simulink model "x12_foc_iden_Jx"  (R2023b)
settings: Solver=VariableStepAuto  StartTime=0.0  StopTime=1  RelTol=1e-3
values from neighbouring files (symbols this model uses):
  Fcoef = 0    [foc_para.m]
  Flux = 0.00525    [foc_para.m]
  id_ki = Rs*CurrentLoopBandwidth    (= 1413.71669412)    [foc_para.m]
  id_kp = Ls*CurrentLoopBandwidth    (= 1.31946891451)    [foc_para.m]
  iq_ki = Rs*CurrentLoopBandwidth    (= 1413.71669412)    [foc_para.m]
  iq_kp = Ls*CurrentLoopBandwidth    (= 1.31946891451)    [foc_para.m]
  iq_limit = 50    [foc_para.m]
  Jx = 0.000004483738    (= 4.483738e-06)    [foc_para.m]
  Ls = 0.00042    [foc_para.m]
  Np = 4    [foc_para.m]
  spd_ki = ((iq_kp/Ls)*(iq_kp/Ls))/(delta*delta*delta*K)    (= 43.9015082323)    [foc_para.m]
  spd_kp = (iq_kp/Ls)/(delta*K)/9.55    (= 0.0234124131329)    [foc_para.m]
  Tpwm = 4000-1    (= 3999)    [foc_para.m]
  Ts = 1/SwitchFrequency    (= 5e-05)    [foc_para.m]
  vbus = 24    [foc_para.m]
  vd_limit = vbus/sqrt(3)    [foc_para.m]
  vq_limit = vbus/sqrt(3)    [foc_para.m]
undefined symbols (not defined in the file or in its folder): DiscIntNeverNeededParam
libraries: spsMosfetLib x6, simulink x3, spsVoltageMeasurementLib x3, spsPermanentMagnetSynchronousMachineLib x1, spsDCVoltageSourceLib x1, sps_lib x1
settings Model: Creator=disnox  LastModifiedBy=disno
settings DataIOCC: ReturnWorkspaceOutputs=off
settings DebuggingCC: ParameterPrecisionLossMsg=none

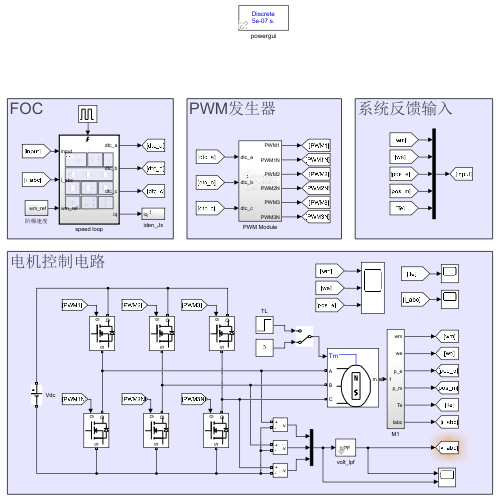
[thumbnail: Simulink's stored preview of the top-level diagram]
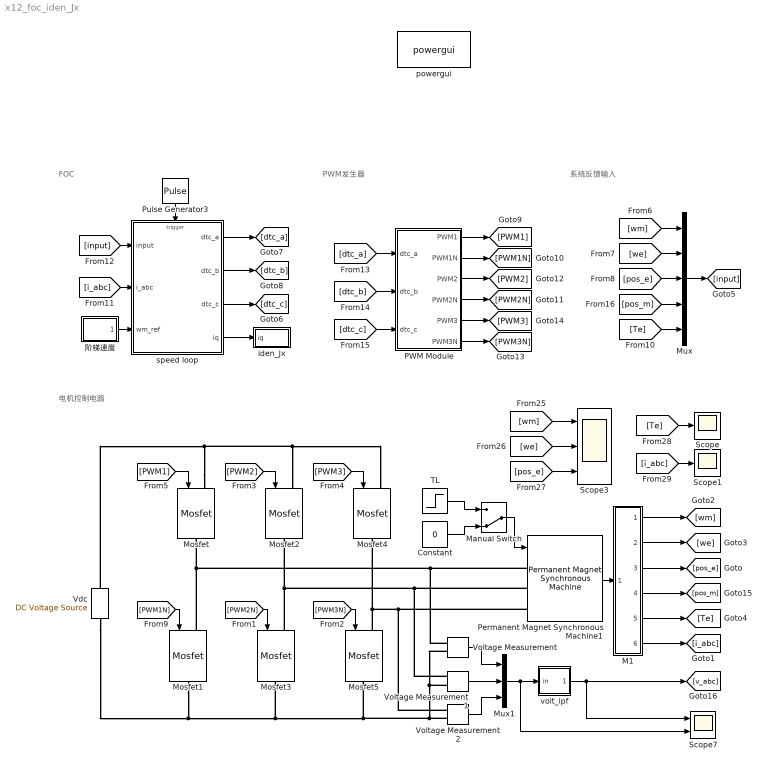
== system x12_foc_iden_Jx ==
  note: FOC
  note: PWM发生器
  note: 系统反馈输入
  note: 电机控制电路
  Constant : Constant  Value=0
  M1 : Subsystem
  Manual Switch : ManualSwitch  CurrentSetting=0
  Mosfet{,1..5} (6 alike) : spsMosfetLib/Mosfet  Ron=0.1  Lon=0  Rd=0.01  Vfd=0  IC=0  Rs=1e5  Cs=inf  Measurements=off
  Mux : Mux  Inputs=5
  Mux1 : Mux  Inputs=3
  PWM Module : Subsystem
  Permanent Magnet Synchronous Machine1 : spsPermanentMagnetSynchronousMachineLib/Permanent Magnet Synchronous Machine  NbPhases=3  FluxDistribution=Sinusoidal  RotorType=Salient-pole  MechanicalLoad=Torque Tm  PresetModel=No  ShowDetailedParameters=on  MeasurementBus=off  Resistance=(Rs)  Inductance=8.5e-3  dqInductances=[Ls, Ls]  La=0.000835  MachineConstant=Flux linkage established by magnets (V.s)  Flux=Flux  VoltageCst=3.809  TorqueCst=0.0315  Flat=120  Mechanical=[Jx Fcoef Np 0]  PolePairs=Np  InitialConditions=[0,0, 0,0]  InitialConditions5ph=[0 0 0 0 0 0]  RefAngle=Aligned with phase A axis (original Park)  IterativeDiscreteModel=Trapezoidal non iterative  TsBlock=-1  TsPowergui=0
  Pulse Generator3 : DiscretePulseGenerator  PulseType=Time based  Period=Ts  PulseWidth=50
  Scope : Scope
  Scope1 : Scope
  Scope3 : Scope  NumInputPorts=3
  Scope7 : Scope  NumInputPorts=2
  TL : Step  Time=0.1  After=0.05  SampleTime=0
  Vdc : spsDCVoltageSourceLib/DC Voltage Source  Amplitude=vbus  Measurements=None
  Voltage Measurement : spsVoltageMeasurementLib/Voltage Measurement  PhasorSimulation=off  OutputType=Complex  PSBequivalent=0
  Voltage Measurement1 : spsVoltageMeasurementLib/Voltage Measurement  PhasorSimulation=off  OutputType=Complex  PSBequivalent=0
  Voltage Measurement2 : spsVoltageMeasurementLib/Voltage Measurement  PhasorSimulation=off  OutputType=Complex  PSBequivalent=0
  iden_Jx : Subsystem
  powergui : sps_lib/powergui  SimulationMode=Discrete  SampleTime=Ts/100  frequency=60  Iterations=50  frequencyindice=0  Pbase=100e6  ErrMax=1e-4  UnitsV=kV  UnitsW=MW  buscounter=0  FunctionMessages=off  echomessages=off  EnableUseOfTLC=off  CurrentSourceSwitches=off  DisableSnubberDevices=off  DisableRonSwitches=off  DisableVfSwitches=off  DisplayEquations=off  AutomaticDiscreteSolvers=off  SolverType=Tustin/Backward Euler (TBE)  Interpol=off  ExternalGateDelay=off  methode=off  Ts=0  x0status=blocks  SPID=off  SwTol=0  HookPort=off  NonlinearTolerance=1e-4  nMaxIteration=100  ContinueOnMaxIteration=off  RestoreLinks=warning  ResistiveCurrentMeasurement=off  Frange=[0:2:500]  Ylog=off  Xlog=on  ShowGrid=off  save=off  variable=ZData  structure=0  ZoomFFT=off  StartTime=0.0  cycles=1  DisplayStyle=1  fundamental=60  FreqAxis=off  MaxFrequency=1000  frequencyindicesteady=1  RmsSteady=1  display=off
  speed loop : Subsystem
  volt_lpf : Subsystem  mask{lpf_freq=1000, Ts=Ts/100}
      mask DialogControl ParameterGroupVar Prompt: 参数
      mask Display: disp('LPF')
  阶梯速度 : Subsystem
  wires:
  Pulse Generator3/1 -> speed loop/Trigger
  [input] -> speed loop/1(input)
  speed loop/2(dtc_b) -> [dtc_b]
  speed loop/1(dtc_a) -> [dtc_a]
  speed loop/3(dtc_c) -> [dtc_c]
  [dtc_a] -> PWM Module/1(dtc_a)
  [dtc_b] -> PWM Module/2(dtc_b)
  [dtc_c] -> PWM Module/3(dtc_c)
  PWM Module/1(PWM1) -> [PWM1]
  PWM Module/2(PWM1N) -> [PWM1N]
  PWM Module/3(PWM2) -> [PWM2]
  PWM Module/4(PWM2N) -> [PWM2N]
  PWM Module/5(PWM3) -> [PWM3]
  PWM Module/6(PWM3N) -> [PWM3N]
  [i_abc] -> speed loop/2(i_abc)
  Mux/1 -> [input]
  [Te] -> Mux/5
  [pos_m] -> Mux/4
  [pos_e] -> Mux/3
  [we] -> Mux/2
  [wm] -> Mux/1
  Manual Switch/1 -> Permanent Magnet Synchronous Machine1/1
  TL/1 -> Manual Switch/1
  [PWM1] -> Mosfet/1
  [PWM2] -> Mosfet2/1
  Constant/1 -> Manual Switch/2
  [PWM2N] -> Mosfet3/1
  Mux1/1 -> Scope7/2, volt_lpf/1(in)
  [PWM3N] -> Mosfet5/1
  M1/1(wm) -> [wm]
  volt_lpf/1(out) -> Scope7/1, [v_abc]
  [PWM3] -> Mosfet4/1
  Voltage Measurement1/1 -> Mux1/2
  [we] -> Scope3/2
  [Te] -> Scope/1
  [pos_e] -> Scope3/3
  Permanent Magnet Synchronous Machine1/1 -> M1/1(In1)
  [wm] -> Scope3/1
  [i_abc] -> Scope1/1
  M1/4(p_m) -> [pos_m]
  Voltage Measurement/1 -> Mux1/1
  M1/6(Iabc) -> [i_abc]
  Voltage Measurement2/1 -> Mux1/3
  [PWM1N] -> Mosfet1/1
  M1/2(we) -> [we]
  M1/3(p_e) -> [pos_e]
  M1/5(Te) -> [Te]
  阶梯速度/1(wm_ref) -> speed loop/3(wm_ref)
  speed loop/4(iq) -> iden_Jx/1(iq)
  connections:
  Voltage Measurement2/LConn1 -- Mosfet5/LConn1 -- Mosfet4/RConn1 -- Permanent Magnet Synchronous Machine1/LConn3
  Mosfet3/RConn1 -- Voltage Measurement2/LConn2 -- Voltage Measurement1/LConn2 -- Voltage Measurement/LConn2 -- Mosfet5/RConn1 -- Vdc/LConn1 -- Mosfet1/RConn1
  Voltage Measurement/LConn1 -- Mosfet1/LConn1 -- Mosfet/RConn1 -- Permanent Magnet Synchronous Machine1/LConn1
  Mosfet/LConn1 -- Mosfet2/LConn1 -- Mosfet4/LConn1 -- Vdc/RConn1
  Mosfet2/RConn1 -- Mosfet3/LConn1 -- Permanent Magnet Synchronous Machine1/LConn2 -- Voltage Measurement1/LConn1

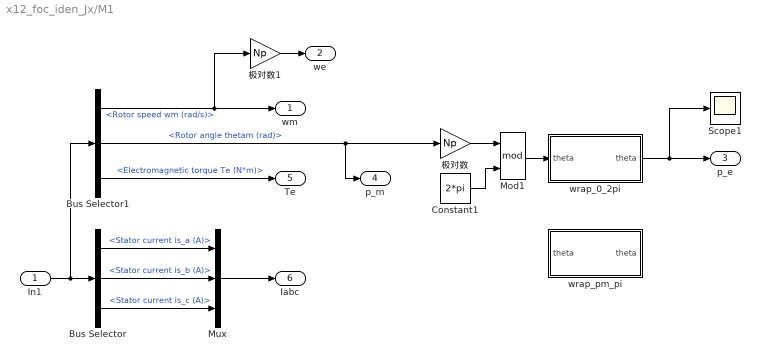
== system x12_foc_iden_Jx/M1 ==
  In1 : Inport
  Bus Selector : BusSelector  OutputSignals=Stator current is_a (A),Stator current is_b (A),Stator current is_c (A)
  Bus Selector1 : BusSelector  OutputSignals=Rotor speed wm (rad/s),Rotor angle thetam (rad),Electromagnetic torque Te (N*m)
  Constant1 : Constant  Value=2*pi
  Mod1 : Math  Operator=mod
  Mux : Mux  Inputs=3
  Scope1 : Scope
  wrap_0_2pi : MATLAB Function  TreatAsAtomicUnit=on
  wrap_pm_pi : MATLAB Function  TreatAsAtomicUnit=on
  极对数 : Gain  Gain=Np
  极对数1 : Gain  Gain=Np
  wm : Outport
  we : Outport  Port=2
  p_e : Outport  Port=3
  p_m : Outport  Port=4
  Te : Outport  Port=5
  Iabc : Outport  Port=6
  wires:
  Bus Selector/1 -> Mux/1  "<Stator current is_a (A)>"
  Bus Selector/2 -> Mux/2  "<Stator current is_b (A)>"
  Bus Selector/3 -> Mux/3  "<Stator current is_c (A)>"
  Bus Selector1/1 -> 极对数1/1, wm/1  "<Rotor speed wm (rad/s)>"
  Bus Selector1/2 -> p_m/1, 极对数/1  "<Rotor angle thetam (rad)>"
  Bus Selector1/3 -> Te/1  "<Electromagnetic torque Te (N*m)>"
  Mux/1 -> Iabc/1
  In1/1 -> Bus Selector1/1, Bus Selector/1
  Constant1/1 -> Mod1/2
  极对数/1 -> Mod1/1
  Mod1/1 -> wrap_0_2pi/1("theta ")
  wrap_0_2pi/1(theta) -> Scope1/1, p_e/1
  极对数1/1 -> we/1

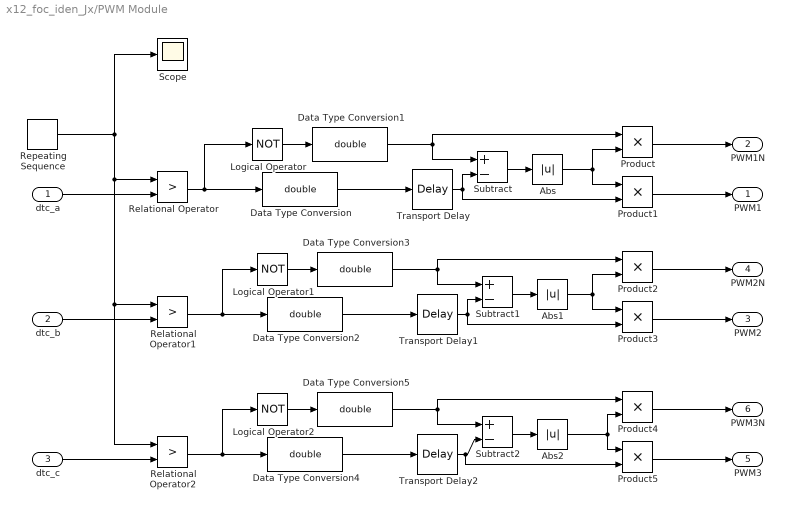
== system x12_foc_iden_Jx/PWM Module ==
  dtc_a : Inport
  dtc_b : Inport  Port=2
  dtc_c : Inport  Port=3
  Abs : Abs  SaturateOnIntegerOverflow=off
  Abs1 : Abs  SaturateOnIntegerOverflow=off
  Abs2 : Abs  SaturateOnIntegerOverflow=off
  Data Type Conversion{,1..5} (6 alike) : DataTypeConversion  OutDataTypeStr=double  SaturateOnIntegerOverflow=off  RndMeth=Floor
  Logical Operator : Logic  Operator=NOT  AllPortsSameDT=off  OutDataTypeStr=boolean
  Logical Operator1 : Logic  Operator=NOT  AllPortsSameDT=off  OutDataTypeStr=boolean
  Logical Operator2 : Logic  Operator=NOT  AllPortsSameDT=off  OutDataTypeStr=boolean
  Product{,1..5} (6 alike) : Product
  Relational Operator : RelationalOperator  Operator=>  OutDataTypeStr=boolean  RndMeth=Simplest  InputSameDT=off
  Relational Operator1 : RelationalOperator  Operator=>  OutDataTypeStr=boolean  RndMeth=Simplest  InputSameDT=off
  Relational Operator2 : RelationalOperator  Operator=>  OutDataTypeStr=boolean  RndMeth=Simplest  InputSameDT=off
  Repeating Sequence : simulink/Sources/Repeating Sequence  rep_seq_t=[0 Ts/2 Ts]  rep_seq_y=[0 Tpwm 0]
  Scope : Scope
  Subtract : Sum  Inputs=+-
  Subtract1 : Sum  Inputs=+-
  Subtract2 : Sum  Inputs=+-
  Transport Delay : TransportDelay  DelayTime=168/168e6
  Transport Delay1 : TransportDelay  DelayTime=168/168e6
  Transport Delay2 : TransportDelay  DelayTime=168/168e6
  PWM1 : Outport
  PWM1N : Outport  Port=2
  PWM2 : Outport  Port=3
  PWM2N : Outport  Port=4
  PWM3 : Outport  Port=5
  PWM3N : Outport  Port=6
  wires:
  Product1/1 -> PWM1/1
  Relational Operator1/1 -> Logical Operator1/1, Data Type Conversion2/1
  Logical Operator2/1 -> Data Type Conversion5/1
  Subtract/1 -> Abs/1
  Relational Operator2/1 -> Data Type Conversion4/1, Logical Operator2/1
  Product4/1 -> PWM3N/1
  Data Type Conversion5/1 -> Subtract2/1, Product4/1
  Product2/1 -> PWM2N/1
  Abs1/1 -> Product2/2, Product3/1
  Transport Delay2/1 -> Subtract2/2, Product5/2
  Repeating Sequence/1 -> Scope/1, Relational Operator/1, Relational Operator2/1, Relational Operator1/1
  Data Type Conversion/1 -> Transport Delay/1
  Product/1 -> PWM1N/1
  Product3/1 -> PWM2/1
  Abs2/1 -> Product5/1, Product4/2
  Data Type Conversion2/1 -> Transport Delay1/1
  dtc_a/1 -> Relational Operator/2
  Transport Delay/1 -> Product1/2, Subtract/2
  Subtract1/1 -> Abs1/1
  Data Type Conversion3/1 -> Subtract1/1, Product2/1
  dtc_c/1 -> Relational Operator2/2
  Logical Operator/1 -> Data Type Conversion1/1
  Transport Delay1/1 -> Product3/2, Subtract1/2
  Relational Operator/1 -> Logical Operator/1, Data Type Conversion/1
  Abs/1 -> Product/2, Product1/1
  Product5/1 -> PWM3/1
  Data Type Conversion4/1 -> Transport Delay2/1
  Subtract2/1 -> Abs2/1
  Logical Operator1/1 -> Data Type Conversion3/1
  Data Type Conversion1/1 -> Subtract/1, Product/1
  dtc_b/1 -> Relational Operator1/2

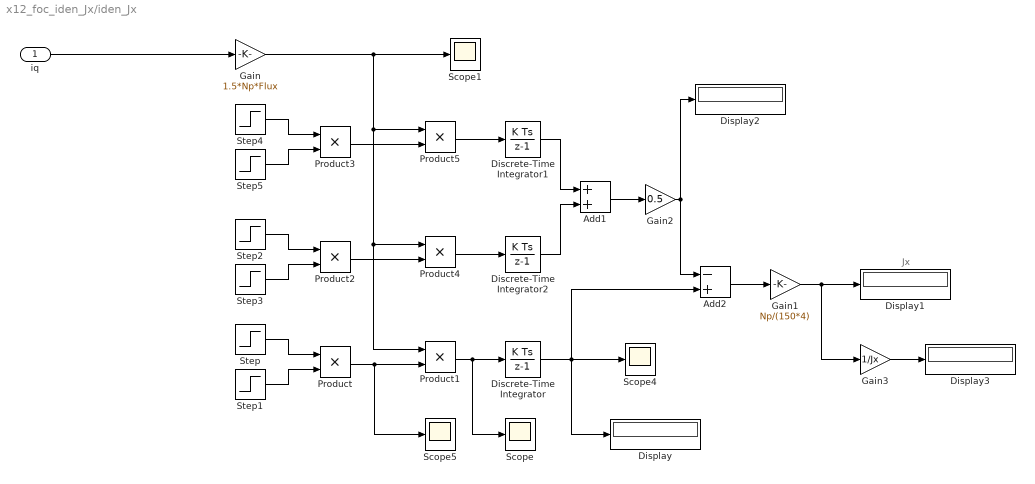
== system x12_foc_iden_Jx/iden_Jx ==
  note: Jx
  iq : Inport
  Add1 : Sum
  Add2 : Sum  Inputs=-+
  Discrete-Time Integrator : DiscreteIntegrator  SampleTime=-1  ICPrevOutput=DiscIntNeverNeededParam  ICPrevScaledInput=DiscIntNeverNeededParam
  Discrete-Time Integrator1 : DiscreteIntegrator  SampleTime=-1  ICPrevOutput=DiscIntNeverNeededParam  ICPrevScaledInput=DiscIntNeverNeededParam
  Discrete-Time Integrator2 : DiscreteIntegrator  SampleTime=-1  ICPrevOutput=DiscIntNeverNeededParam  ICPrevScaledInput=DiscIntNeverNeededParam
  Display{,1..3} (4 alike) : Display
  Gain : Gain  Gain=1.5*Np*Flux
  Gain1 : Gain  Gain=Np/(150*4)
  Gain2 : Gain  Gain=0.5
  Gain3 : Gain  Gain=1/Jx
  Product{,1..5} (6 alike) : Product
  Scope{,1,4..5} (4 alike) : Scope
  Step : Step  Time=0.65  SampleTime=0
  Step1 : Step  Time=0.8  Before=1  After=0  SampleTime=0
  Step2 : Step  Time=0.83  SampleTime=0
  Step3 : Step  Time=0.98  Before=1  After=0  SampleTime=0
  Step4 : Step  Time=0.42  SampleTime=0
  Step5 : Step  Time=0.57  Before=1  After=0  SampleTime=0
  wires:
  Step4/1 -> Product3/1
  Product/1 -> Scope5/1, Product1/2
  Product3/1 -> Product5/2
  Gain/1 -> Scope1/1, Product5/1, Product4/1, Product1/1
  Step1/1 -> Product/2
  Product1/1 -> Scope/1, Discrete-Time Integrator/1
  Product2/1 -> Product4/2
  Gain2/1 -> Display2/1, Add2/1
  Step/1 -> Product/1
  Discrete-Time Integrator1/1 -> Add1/1
  Step5/1 -> Product3/2
  Step3/1 -> Product2/2
  Discrete-Time Integrator/1 -> Scope4/1, Display/1, Add2/2
  Step2/1 -> Product2/1
  Product5/1 -> Discrete-Time Integrator1/1
  Add1/1 -> Gain2/1
  Discrete-Time Integrator2/1 -> Add1/2
  Add2/1 -> Gain1/1
  Gain1/1 -> Gain3/1, Display1/1
  Product4/1 -> Discrete-Time Integrator2/1
  iq/1 -> Gain/1
  Gain3/1 -> Display3/1

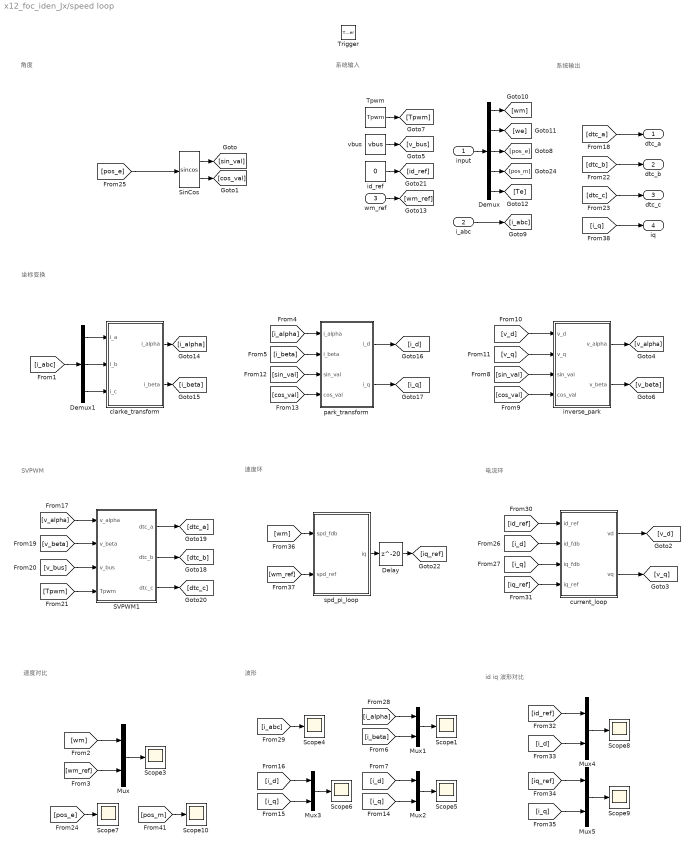
== system x12_foc_iden_Jx/speed loop ==
  note: 角度
  note: 坐标变换
  note: SVPWM
  note: 速度对比
  note: 波形
  note: 系统输入
  note: 系统输出
  note: 电流环
  note: id iq 波形对比
  note: 速度环
  input : Inport
  i_abc : Inport  Port=2
  wm_ref : Inport  Port=3
  Trigger : TriggerPort  VariantControl=(inherit)
  Delay : Delay  DelayLength=20
  Demux : Demux  Outputs=5
  Demux1 : Demux  Outputs=3
  Mux{,1..5} (6 alike) : Mux  Inputs=2
  SVPWM1 : Subsystem  TreatAsAtomicUnit=on
      settings: RTWSystemCode=Nonreusable function  RTWFcnNameOpts=Use subsystem name
  Scope{1,3..10} (9 alike) : Scope
  SinCos : Trigonometry  Operator=sincos
  Tpwm : Constant  Value=Tpwm
  clarke_transform : Subsystem  TreatAsAtomicUnit=on
      settings: RTWSystemCode=Nonreusable function  RTWFcnNameOpts=Use subsystem name
  current_loop : Subsystem
  id_ref : Constant  Value=0
  inverse_park : Subsystem  TreatAsAtomicUnit=on
      settings: RTWSystemCode=Nonreusable function  RTWFcnNameOpts=Use subsystem name
  park_transform : Subsystem  TreatAsAtomicUnit=on
      settings: RTWSystemCode=Nonreusable function  RTWFcnNameOpts=Use subsystem name
  spd_pi_loop : Subsystem  TreatAsAtomicUnit=on
      settings: RTWSystemCode=Nonreusable function  RTWFcnNameOpts=Use subsystem name
  vbus : Constant  Value=vbus
  dtc_a : Outport
  dtc_b : Outport  Port=2
  dtc_c : Outport  Port=3
  iq : Outport  Port=4
  wires:
  SinCos/1 -> [sin_val]
  SinCos/2 -> [cos_val]
  wm_ref/1 -> [wm_ref]
  id_ref/1 -> [id_ref]
  [cos_val] -> inverse_park/4(cos_val)
  [sin_val] -> park_transform/3(sin_val)
  [v_d] -> inverse_park/1(v_d)
  [v_q] -> inverse_park/2(v_q)
  [cos_val] -> park_transform/4(cos_val)
  [sin_val] -> inverse_park/3(sin_val)
  [v_beta] -> SVPWM1/2(v_beta)
  [v_alpha] -> SVPWM1/1(v_alpha)
  [Tpwm] -> SVPWM1/4(Tpwm)
  [v_bus] -> SVPWM1/3(v_bus)
  Tpwm/1 -> [Tpwm]
  vbus/1 -> [v_bus]
  inverse_park/2(v_beta) -> [v_beta]
  inverse_park/1(v_alpha) -> [v_alpha]
  Demux1/1 -> clarke_transform/1(i_a)
  Demux1/2 -> clarke_transform/2(i_b)
  Demux1/3 -> clarke_transform/3(i_c)
  [i_abc] -> Demux1/1
  [wm] -> Mux/1
  [wm_ref] -> Mux/2
  Mux/1 -> Scope3/1
  i_abc/1 -> [i_abc]
  [i_alpha] -> park_transform/1(i_alpha)
  [i_beta] -> park_transform/2(i_beta)
  clarke_transform/1(i_alpha) -> [i_alpha]
  clarke_transform/2(i_beta) -> [i_beta]
  park_transform/1(i_d) -> [i_d]
  park_transform/2(i_q) -> [i_q]
  [i_abc] -> Scope4/1
  [i_alpha] -> Mux1/1
  Mux1/1 -> Scope1/1
  [i_beta] -> Mux1/2
  [i_q] -> Mux2/2
  [i_d] -> Mux2/1
  Mux2/1 -> Scope5/1
  [i_d] -> Mux3/1
  Mux3/1 -> Scope6/1
  [i_q] -> Mux3/2
  [dtc_b] -> dtc_b/1
  [dtc_c] -> dtc_c/1
  [dtc_a] -> dtc_a/1
  SVPWM1/3(dtc_c) -> [dtc_c]
  SVPWM1/2(dtc_b) -> [dtc_b]
  SVPWM1/1(dtc_a) -> [dtc_a]
  [pos_e] -> SinCos/1
  [pos_e] -> Scope7/1
  [i_d] -> current_loop/2(id_fdb)
  [i_q] -> current_loop/3(iq_fdb)
  current_loop/1(vd) -> [v_d]
  current_loop/2(vq) -> [v_q]
  [iq_ref] -> current_loop/4(iq_ref)
  [id_ref] -> current_loop/1(id_ref)
  [id_ref] -> Mux4/1
  Mux4/1 -> Scope8/1
  [i_d] -> Mux4/2
  [iq_ref] -> Mux5/1
  Mux5/1 -> Scope9/1
  [i_q] -> Mux5/2
  spd_pi_loop/1(iq) -> Delay/1
  Delay/1 -> [iq_ref]
  [wm] -> spd_pi_loop/1(spd_fdb)
  [wm_ref] -> spd_pi_loop/2(spd_ref)
  [pos_m] -> Scope10/1
  Demux/3 -> [pos_e]
  Demux/5 -> [Te]
  Demux/2 -> [we]
  Demux/4 -> [pos_m]
  input/1 -> Demux/1
  Demux/1 -> [wm]
  [i_q] -> iq/1

== system x12_foc_iden_Jx/volt_lpf ==
  in : Inport
  Add : Sum
  Constant2 : Constant  Value=1-(1/(1+lpf_freq*6.28*Ts))
  Constant3 : Constant  Value=1/(1+lpf_freq*6.28*Ts)
  Product1 : Product
  Product2 : Product
  Unit Delay1 : UnitDelay  SampleTime=-1  HasFrameUpgradeWarning=on
  out : Outport
  wires:
  Constant3/1 -> Product2/1
  Constant2/1 -> Product1/1
  Product1/1 -> Add/1
  Unit Delay1/1 -> Product2/2
  Add/1 -> out/1, Unit Delay1/1
  Product2/1 -> Add/2
  in/1 -> Product1/2

== system x12_foc_iden_Jx/阶梯速度 ==
  Add : Sum
  Ramp1 : simulink/Sources/Ramp  slope=1000  start=0  InitialOutput=0
  Ramp2 : simulink/Sources/Ramp  slope=1000  start=0.6  InitialOutput=0
  Saturation : Saturate  UpperLimit=400
  Saturation1 : Saturate  UpperLimit=200
  wm_ref : Outport
  wires:
  Ramp2/1 -> Saturation1/1
  Saturation1/1 -> Add/2
  Saturation/1 -> Add/1
  Ramp1/1 -> Saturation/1
  Add/1 -> wm_ref/1

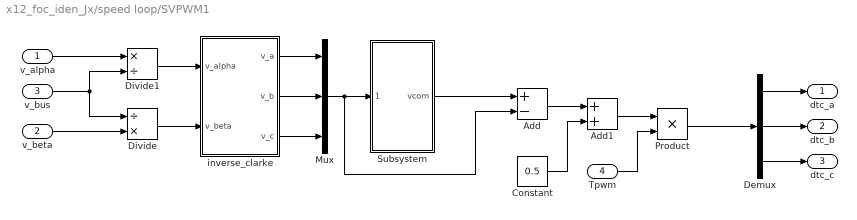
== system x12_foc_iden_Jx/speed loop/SVPWM1 ==
  v_alpha : Inport
  v_beta : Inport  Port=2
  v_bus : Inport  Port=3
  Tpwm : Inport  Port=4
  Add : Sum  Inputs=+-
  Add1 : Sum
  Constant : Constant  Value=0.5
  Demux : Demux  Outputs=3
  Divide : Product  Inputs=/*
  Divide1 : Product  Inputs=*/
  Mux : Mux  Inputs=3
  Product : Product
  Subsystem : Subsystem
  inverse_clarke : Subsystem  TreatAsAtomicUnit=on
      settings: RTWSystemCode=Nonreusable function  RTWFcnNameOpts=Use subsystem name
  dtc_a : Outport
  dtc_b : Outport  Port=2
  dtc_c : Outport  Port=3
  wires:
  Demux/1 -> dtc_a/1
  Demux/2 -> dtc_b/1
  Demux/3 -> dtc_c/1
  inverse_clarke/2(v_b) -> Mux/2
  inverse_clarke/1(v_a) -> Mux/1
  inverse_clarke/3(v_c) -> Mux/3
  Mux/1 -> Subsystem/1(v_abc), Add/2
  Subsystem/1(vcom) -> Add/1
  Add/1 -> Add1/1
  Constant/1 -> Add1/2
  Add1/1 -> Product/1
  Product/1 -> Demux/1
  Tpwm/1 -> Product/2
  Divide/1 -> inverse_clarke/2(v_beta)
  Divide1/1 -> inverse_clarke/1(v_alpha)
  v_alpha/1 -> Divide1/1
  v_beta/1 -> Divide/2
  v_bus/1 -> Divide/1, Divide1/2

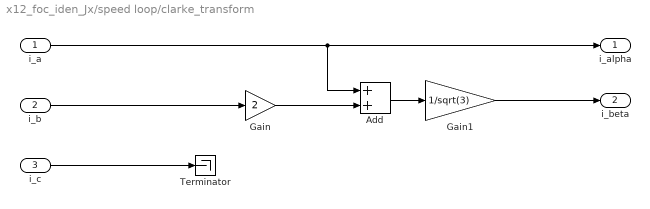
== system x12_foc_iden_Jx/speed loop/clarke_transform ==
  i_a : Inport
  i_b : Inport  Port=2
  i_c : Inport  Port=3
  Add : Sum
  Gain : Gain  Gain=2
  Gain1 : Gain  Gain=1/sqrt(3)
  Terminator : Terminator
  i_alpha : Outport
  i_beta : Outport  Port=2
  wires:
  i_a/1 -> Add/1, i_alpha/1
  i_b/1 -> Gain/1
  Gain/1 -> Add/2
  Add/1 -> Gain1/1
  Gain1/1 -> i_beta/1
  i_c/1 -> Terminator/1

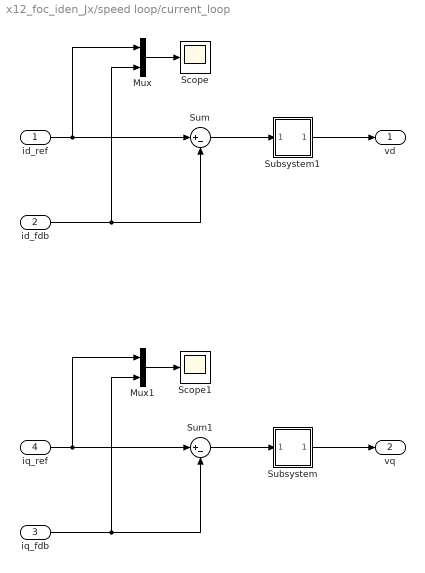
== system x12_foc_iden_Jx/speed loop/current_loop ==
  id_ref : Inport
  id_fdb : Inport  Port=2
  iq_fdb : Inport  Port=3
  iq_ref : Inport  Port=4
  Mux : Mux  Inputs=2
  Mux1 : Mux  Inputs=2
  Scope : Scope
  Scope1 : Scope
  Subsystem : Subsystem  mask{kp=iq_kp, ki=iq_ki, limit=vq_limit}
      mask DialogControl PI Prompt: PI
      mask DialogControl ParameterGroupVar Prompt: 参数
      mask Display: disp('PI')
  Subsystem1 : Subsystem  mask{kp=id_kp, ki=id_ki, limit=vd_limit}
      mask DialogControl PI Prompt: PI
      mask DialogControl ParameterGroupVar Prompt: 参数
      mask Display: disp('PI')
  Sum : Sum  Inputs=|+-
  Sum1 : Sum  Inputs=|+-
  vd : Outport
  vq : Outport  Port=2
  wires:
  id_fdb/1 -> Mux/2, Sum/2
  Mux/1 -> Scope/1
  id_ref/1 -> Mux/1, Sum/1
  iq_ref/1 -> Mux1/1, Sum1/1
  Mux1/1 -> Scope1/1
  iq_fdb/1 -> Mux1/2, Sum1/2
  Sum1/1 -> Subsystem/1(error)
  Subsystem/1(Out1) -> vq/1
  Sum/1 -> Subsystem1/1(error)
  Subsystem1/1(Out1) -> vd/1

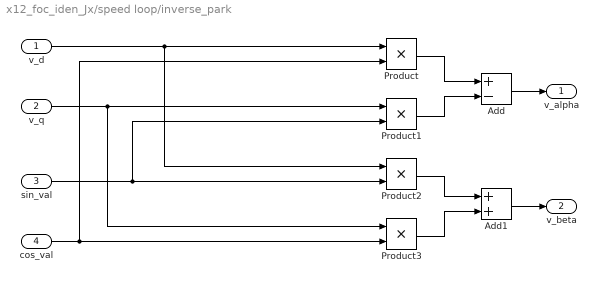
== system x12_foc_iden_Jx/speed loop/inverse_park ==
  v_d : Inport
  v_q : Inport  Port=2
  sin_val : Inport  Port=3
  cos_val : Inport  Port=4
  Add : Sum  Inputs=+-
  Add1 : Sum  AccumDataTypeStr=double
  Product{,1..3} (4 alike) : Product
  v_alpha : Outport
  v_beta : Outport  Port=2
  wires:
  v_d/1 -> Product2/1, Product/1
  cos_val/1 -> Product3/2, Product/2
  Product/1 -> Add/1
  Product1/1 -> Add/2
  v_q/1 -> Product1/1, Product3/1
  sin_val/1 -> Product2/2, Product1/2
  Add/1 -> v_alpha/1
  Product2/1 -> Add1/1
  Product3/1 -> Add1/2
  Add1/1 -> v_beta/1

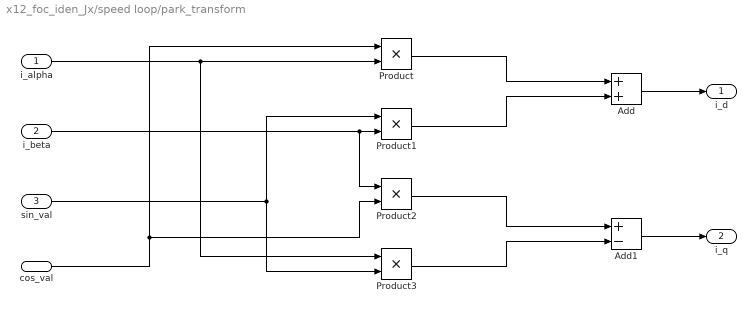
== system x12_foc_iden_Jx/speed loop/park_transform ==
  i_alpha : Inport
  i_beta : Inport  Port=2
  sin_val : Inport  Port=3
  cos_val : Inport  Port=4
  Add : Sum
  Add1 : Sum  Inputs=+-
  Product{,1..3} (4 alike) : Product
  i_d : Outport
  i_q : Outport  Port=2
  wires:
  i_alpha/1 -> Product/2, Product3/1
  cos_val/1 -> Product2/2, Product/1
  sin_val/1 -> Product3/2, Product1/1
  i_beta/1 -> Product2/1, Product1/2
  Product/1 -> Add/1
  Product1/1 -> Add/2
  Add/1 -> i_d/1
  Product2/1 -> Add1/1
  Product3/1 -> Add1/2
  Add1/1 -> i_q/1

== system x12_foc_iden_Jx/speed loop/spd_pi_loop ==
  spd_fdb : Inport
  spd_ref : Inport  Port=2
  Mux : Mux  Inputs=2
  Scope : Scope
  Subsystem : Subsystem  mask{kp=spd_kp, ki=spd_ki, limit=iq_limit}
      mask DialogControl PI Prompt: PI
      mask DialogControl ParameterGroupVar Prompt: 参数
      mask Display: disp('PI')
  Sum : Sum  Inputs=|+-
  iq : Outport
  wires:
  spd_ref/1 -> Mux/1, Sum/1
  spd_fdb/1 -> Mux/2, Sum/2
  Mux/1 -> Scope/1
  Sum/1 -> Subsystem/1(error)
  Subsystem/1(Out1) -> iq/1

== system x12_foc_iden_Jx/speed loop/SVPWM1/Subsystem ==
  v_abc : Inport
  Add : Sum
  Demux : Demux  Outputs=3
  Gain : Gain  Gain=0.5
  Max : MinMax  Function=max  Inputs=3
  Min : MinMax  Inputs=3
  vcom : Outport
  wires:
  Min/1 -> Add/1
  Max/1 -> Add/2
  Add/1 -> Gain/1
  Gain/1 -> vcom/1
  Demux/1 -> Max/1, Min/1
  Demux/2 -> Max/2, Min/2
  Demux/3 -> Max/3, Min/3
  v_abc/1 -> Demux/1

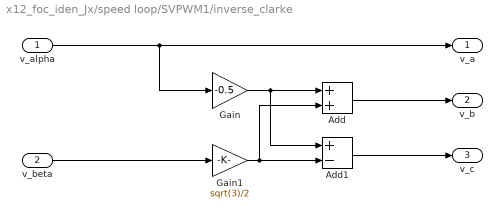
== system x12_foc_iden_Jx/speed loop/SVPWM1/inverse_clarke ==
  v_alpha : Inport
  v_beta : Inport  Port=2
  Add : Sum
  Add1 : Sum  Inputs=+-
  Gain : Gain  Gain=-0.5
  Gain1 : Gain  Gain=sqrt(3)/2
  v_a : Outport
  v_b : Outport  Port=2
  v_c : Outport  Port=3
  wires:
  v_alpha/1 -> Gain/1, v_a/1
  Gain/1 -> Add1/1, Add/1
  v_beta/1 -> Gain1/1
  Gain1/1 -> Add/2, Add1/2
  Add/1 -> v_b/1
  Add1/1 -> v_c/1

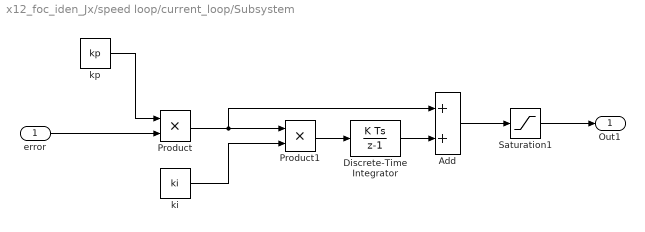
== system x12_foc_iden_Jx/speed loop/current_loop/Subsystem ==
  error : Inport
  Add : Sum
  Discrete-Time Integrator : DiscreteIntegrator  SampleTime=-1  LimitOutput=on  UpperSaturationLimit=vq_limit  LowerSaturationLimit=-vq_limit  ICPrevOutput=DiscIntNeverNeededParam  ICPrevScaledInput=DiscIntNeverNeededParam
  Product : Product
  Product1 : Product
  Saturation1 : Saturate  UpperLimit=limit  LowerLimit=-limit
  ki : Constant  Value=ki  OutDataTypeStr=single
  kp : Constant  Value=kp  VectorParams1D=off  OutDataTypeStr=single
  Out1 : Outport
  wires:
  Product1/1 -> Discrete-Time Integrator/1
  Discrete-Time Integrator/1 -> Add/2
  Product/1 -> Add/1, Product1/1
  kp/1 -> Product/1
  ki/1 -> Product1/2
  Saturation1/1 -> Out1/1
  Add/1 -> Saturation1/1
  error/1 -> Product/2

== system x12_foc_iden_Jx/speed loop/current_loop/Subsystem1 ==
  error : Inport
  Add : Sum
  Discrete-Time Integrator : DiscreteIntegrator  SampleTime=-1  LimitOutput=on  UpperSaturationLimit=vd_limit  LowerSaturationLimit=-vd_limit  ICPrevOutput=DiscIntNeverNeededParam  ICPrevScaledInput=DiscIntNeverNeededParam
  Product : Product
  Product1 : Product
  Saturation1 : Saturate  UpperLimit=limit  LowerLimit=-limit
  ki : Constant  Value=ki  OutDataTypeStr=single
  kp : Constant  Value=kp  VectorParams1D=off  OutDataTypeStr=single
  Out1 : Outport
  wires:
  Product1/1 -> Discrete-Time Integrator/1
  Discrete-Time Integrator/1 -> Add/2
  Product/1 -> Add/1, Product1/1
  kp/1 -> Product/1
  ki/1 -> Product1/2
  Saturation1/1 -> Out1/1
  Add/1 -> Saturation1/1
  error/1 -> Product/2

== system x12_foc_iden_Jx/speed loop/spd_pi_loop/Subsystem ==
  error : Inport
  Add : Sum
  Discrete-Time Integrator : DiscreteIntegrator  SampleTime=-1  LimitOutput=on  UpperSaturationLimit=iq_limit  LowerSaturationLimit=-iq_limit  ICPrevOutput=DiscIntNeverNeededParam  ICPrevScaledInput=DiscIntNeverNeededParam
  Product : Product
  Product1 : Product
  Saturation1 : Saturate  UpperLimit=limit  LowerLimit=-limit
  ki : Constant  Value=ki  OutDataTypeStr=single
  kp : Constant  Value=kp  VectorParams1D=off  OutDataTypeStr=single
  Out1 : Outport
  wires:
  Product1/1 -> Discrete-Time Integrator/1
  Discrete-Time Integrator/1 -> Add/2
  Product/1 -> Add/1, Product1/1
  kp/1 -> Product/1
  ki/1 -> Product1/2
  Saturation1/1 -> Out1/1
  Add/1 -> Saturation1/1
  error/1 -> Product/2

== matlab function x12_foc_iden_Jx/M1/wrap_pm_pi ==
  data: theta output; theta input
function theta = wrap_pm_pi(theta)

    M_PI = pi;
    M_2PI = 2*pi;
    
    if theta > M_PI
        theta = theta - M_2PI;
    elseif theta < -M_PI
        theta = theta + M_2PI;
    end
end

== matlab function x12_foc_iden_Jx/M1/wrap_0_2pi ==
  data: theta output; theta input
function theta = wrap_0_2pi(theta)

    M_2PI = 2*pi;
    
    if theta > M_2PI
        theta = theta - M_2PI;
    elseif theta < 0
        theta = theta + M_2PI;
    end
end
